simulink model "casestudy1"  (Simulink 8.5)
settings: Solver=ode45  StartTime=0.0  StopTime=10  RelTol=1e-3
values from neighbouring files (symbols this model uses):
  Z0 = [pi/4;-pi/4;0;0]    [setup.m]
undefined symbols (not defined in the file or in its folder): case_invkin, extforce, forward_kin_2link, IJSMC, stateder
settings Model: Creator=rhanz  LastModifiedBy=rhanz  ExtModeAutoUpdateStatusClock=off
settings OptimizationCC: InitFltsAndDblsToZero=on
settings DebuggingCC: SaveWithParameterizedLinksMsg=none  SignalResolutionControl=TryResolveAllWithWarning  SolverPrmCheckMsg=warning  MultiTaskDSMMsg=warning  MultiTaskCondExecSysMsg=none  FcnCallInpInsideContextMsg=UseLocalSettings
settings GRTTargetCC: TargetFcnLib=ansi_tfl_tmw.mat

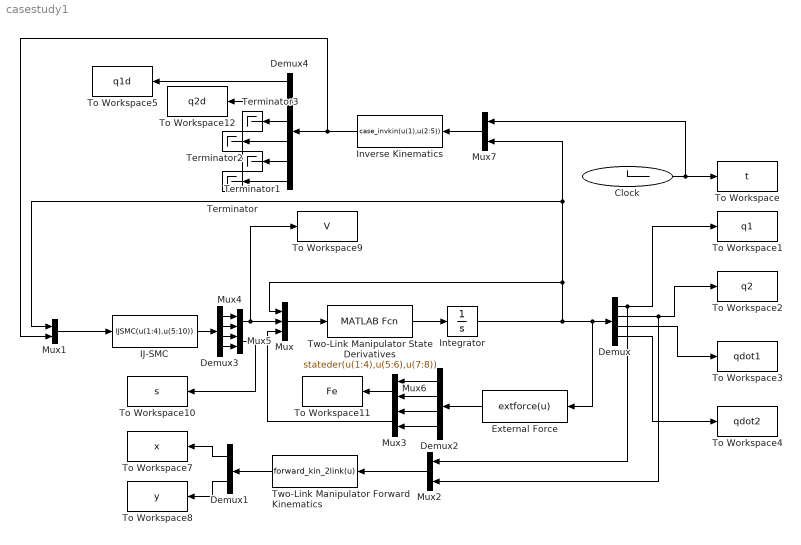
== system casestudy1 ==
  Clock : Clock
  Demux : Demux
  Demux1 : Demux  Outputs=2
  Demux2 : Demux
  Demux3 : Demux
  Demux4 : Demux  Outputs=6
  External Force : MATLABFcn  MATLABFcn=extforce(u)  OutputDimensions=4
  IJ-SMC : MATLABFcn  MATLABFcn=IJSMC(u(1:4),u(5:10))  OutputDimensions=4
  Integrator : Integrator  InitialCondition=Z0
  Inverse Kinematics : MATLABFcn  MATLABFcn=case_invkin(u(1),u(2:5))  OutputDimensions=6
  Mux : Mux  Inputs=3
  Mux{1..7} (7 alike) : Mux  Inputs=2
  Terminator{,1..3} (4 alike) : Terminator
  To Workspace : ToWorkspace  VariableName=t  SampleTime=-1
  To Workspace1 : ToWorkspace  VariableName=q1  SampleTime=-1
  To Workspace10 : ToWorkspace  VariableName=s  SampleTime=-1
  To Workspace11 : ToWorkspace  VariableName=Fe  SampleTime=-1
  To Workspace12 : ToWorkspace  VariableName=q2d  SampleTime=-1
  To Workspace2 : ToWorkspace  VariableName=q2  SampleTime=-1
  To Workspace3 : ToWorkspace  VariableName=qdot1  SampleTime=-1
  To Workspace4 : ToWorkspace  VariableName=qdot2  SampleTime=-1
  To Workspace5 : ToWorkspace  VariableName=q1d  SampleTime=-1
  To Workspace7 : ToWorkspace  VariableName=x  SampleTime=-1
  To Workspace8 : ToWorkspace  VariableName=y  SampleTime=-1
  To Workspace9 : ToWorkspace  VariableName=V  SampleTime=-1
  Two-Link Manipulator Forward Kinematics : MATLABFcn  MATLABFcn=forward_kin_2link(u)  OutputDimensions=2
  Two-Link Manipulator State Derivatives : MATLABFcn  MATLABFcn=stateder(u(1:4),u(5:6),u(7:8))  OutputDimensions=4
  wires:
  Two-Link Manipulator State Derivatives/1 -> Integrator/1
  Mux/1 -> Two-Link Manipulator State Derivatives/1
  Clock/1 -> Mux7/1, To Workspace/1
  Demux/1 -> To Workspace1/1, Mux2/1
  Demux/4 -> To Workspace4/1
  Mux2/1 -> Two-Link Manipulator Forward Kinematics/1
  Demux1/1 -> To Workspace7/1
  Demux1/2 -> To Workspace8/1
  Two-Link Manipulator Forward Kinematics/1 -> Demux1/1
  External Force/1 -> Demux2/1
  Demux2/3 -> Mux3/1
  Demux2/4 -> Mux3/2
  Mux3/1 -> Mux/3
  IJ-SMC/1 -> Demux3/1
  Mux4/1 -> To Workspace9/1, Mux/2
  Demux3/1 -> Mux4/1
  Demux3/2 -> Mux4/2
  Demux3/3 -> Mux5/1
  Demux3/4 -> Mux5/2
  Mux5/1 -> To Workspace10/1
  Demux/3 -> To Workspace3/1
  Demux/2 -> Mux2/2, To Workspace2/1
  Demux2/1 -> Mux6/1
  Demux2/2 -> Mux6/2
  Mux6/1 -> To Workspace11/1
  Demux4/6 -> Terminator/1
  Demux4/5 -> Terminator1/1
  Demux4/4 -> Terminator2/1
  Demux4/3 -> Terminator3/1
  Demux4/1 -> To Workspace5/1
  Demux4/2 -> To Workspace12/1
  Mux1/1 -> IJ-SMC/1
  Inverse Kinematics/1 -> Mux1/2, Demux4/1
  Mux7/1 -> Inverse Kinematics/1
  Integrator/1 -> External Force/1, Demux/1, Mux/1, Mux7/2, Mux1/1
